simulink model "Joystick_ReadAndSend_X3D"  (R2017a)
settings: Solver=FixedStepAuto  StartTime=0.0  StopTime=inf  FixedStep=0.01  RelTol=1e-3
undefined symbols (not defined in the file or in its folder): Joystick, Standard_Devices, UDP_Protocol
libraries: sldrtlib x3
settings Model: Creator=kivela6  LastModifiedBy=aha

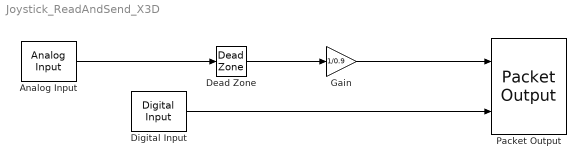
== system Joystick_ReadAndSend_X3D ==
  Analog Input : sldrtlib/Analog Input  SampleTime=0.01  MaxMissedTicks=1000  ShowMissedTicks=off  YieldWhenWaiting=off  DrvName=Standard_Devices/Joystick  DrvAddress=1  DrvOptions=zeros(1,0)  Channels=[1:4]  RangeMode=2  VoltRange=1  DataType=1
      settings: AttributesFormatString=Standard Devices\nJoystick [1h]  SourceProductName=Simulink Desktop Real-Time
  Dead Zone : DeadZone  LowerValue=-0.1  UpperValue=0.1  SaturateOnIntegerOverflow=on
  Digital Input : sldrtlib/Digital Input  SampleTime=0.01  MaxMissedTicks=1000  ShowMissedTicks=off  YieldWhenWaiting=off  DrvName=Standard_Devices/Joystick  DrvAddress=1  DrvOptions=zeros(1,0)  Channels=[1:12]  BitMode=1  DataType=4
      settings: AttributesFormatString=Standard Devices\nJoystick [1h]  SourceProductName=Simulink Desktop Real-Time  SourceProductBaseCode=WT
  Gain : Gain  Gain=1/0.9
  Packet Output : sldrtlib/Packet Output  SampleTime=0.01  MaxMissedTicks=1000  ShowMissedTicks=off  YieldWhenWaiting=off  DrvName=Standard_Devices/UDP_Protocol  DrvAddress=12000  DrvOptions=[3232238082 55550]  PacketSize=44  DataTypes={'4*double','12*uint8'}  ShowReady=off  ShowError=off  PacketID=1  ByteOrder=1  InitialValue=[]  FinalValue=[]
      settings: AttributesFormatString=Standard Devices\nUDP Protocol [2EE0h]  SourceProductName=Simulink Desktop Real-Time
  wires:
  Digital Input/1 -> Packet Output/2
  Analog Input/1 -> Dead Zone/1
  Dead Zone/1 -> Gain/1
  Gain/1 -> Packet Output/1
